simulink model "BlsmControl_color"  (R2014a)
settings: Solver=FixedStepDiscrete  SolverMode=SingleTasking  StartTime=0.0  StopTime=6  FixedStep=1e-4  MinStep=1e-7  RelTol=1e-4  AbsTol=1e-4
PostLoadFcn:
  | parameter
InitFcn:
  | parameter
undefined symbols (not defined in the file): PI, rpm_ast
libraries: simulink x1
settings Model: CovSFcnEnable=on  ExtModeTrigDuration=100  BufferReuse=off  Creator=matsumoto  LastModifiedBy=ts1413
settings DataIOCC: SaveFinalState=on  SignalLoggingSaveFormat=ModelDataLogs  SaveOutput=off  SaveState=on  StateSaveName=tmp_raccel_xout  SignalLoggingName=tmp_raccel_logsout
settings OptimizationCC: BlockReduction=off  OptimizeBlockIOStorage=off  BufferReuse=off  GlobalBufferReuse=off  ExpressionFolding=off  ExpressionDepthLimit=2147483647  LocalBlockOutputs=off  EfficientMapNaN2IntZero=off  OptimizeModelRefInitCode=on  LifeSpan=1
settings DebuggingCC: ConsistencyChecking=warning  UnderspecifiedInitializationDetection=Classic  TimeAdjustmentMsg=warning  FcnCallInpInsideContextMsg=UseLocalSettings  FrameProcessingCompatibilityMsg=error  StateNameClashWarn=warning
settings HardwareCC: TargetBitPerLong=64  TargetBitPerPointer=64  TargetLongLongMode=on  TargetIntDivRoundTo=Zero  TargetEndianess=LittleEndian  TargetWordSize=64  TargetHWDeviceType=MATLAB Host  ProdEqTarget=off
settings RTWCC: SystemTargetFile=ert.tlc  GenCodeOnly=on  TemplateMakefile=ert_default_tmf  Description=Embedded Coder  ProcessScript=ert_make_rtw_hook
settings CodeAppCC: IgnoreCustomStorageClasses=off  MaxIdLength=128
settings ERTTargetCC: ParMdlRefBuildCompliant=on  CompOptLevelCompliant=on  ConcurrentExecutionCompliant=on  ERTFirstTimeCompliant=on  ModelStepFunctionPrototypeControlCompliant=on  CPPClassGenCompliant=on  InlinedParameterPlacement=Hierarchical  ERTCustomFileTemplate=example_file_process.tlc
settings ConfigComp: CovMetricSettings=dw  CovHtmlReporting=on  CovSaveCumulativeToWorkspaceVar=on  CovSaveSingleToWorkspaceVar=on  CovModelRefEnable=Off  CovExternalEMLEnable=off

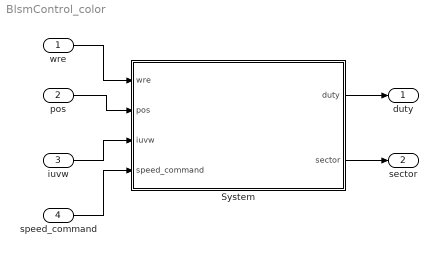
== system BlsmControl_color ==
  wre : Inport
  pos : Inport  Port=2
  iuvw : Inport  Port=3
  speed_command : Inport  Port=4
  System : Subsystem
  duty : Outport
  sector : Outport  Port=2
  wires:
  wre/1 -> System/1(wre)
  pos/1 -> System/2(pos)
  iuvw/1 -> System/3(iuvw)
  speed_command/1 -> System/4(speed_command)
  System/1(duty) -> duty/1
  System/2(sector) -> sector/1

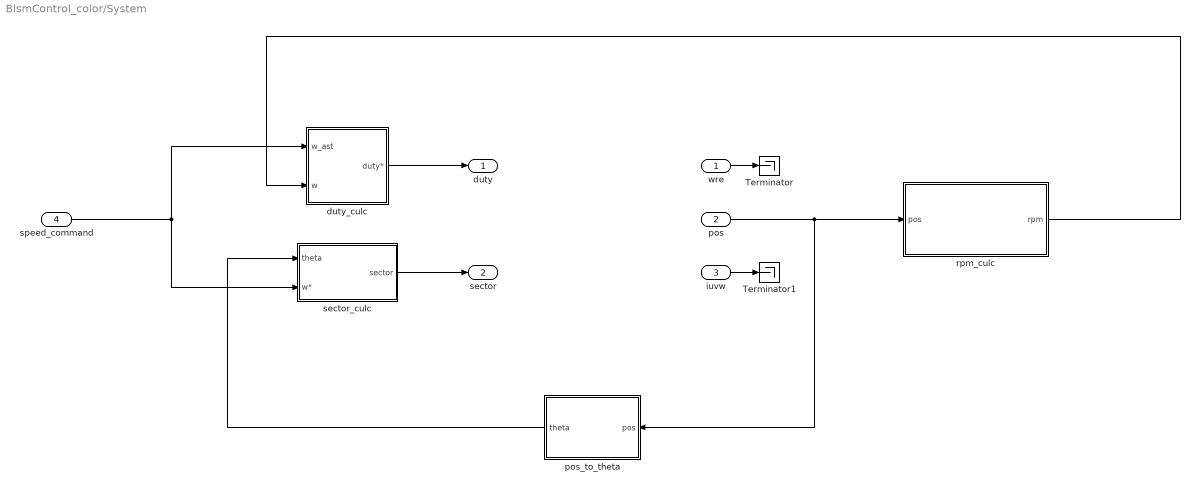
== system BlsmControl_color/System ==
  wre : Inport
  pos : Inport  Port=2
  iuvw : Inport  Port=3
  speed_command : Inport  Port=4
  Terminator : Terminator
  Terminator1 : Terminator
  duty_culc : Subsystem
  pos_to_theta : Subsystem
  rpm_culc : Subsystem
  sector_culc : Subsystem
  duty : Outport
  sector : Outport  Port=2
  wires:
  sector_culc/1(sector) -> sector/1
  pos/1 -> rpm_culc/1(pos), pos_to_theta/1(pos)
  duty_culc/1(duty*) -> duty/1
  speed_command/1 -> duty_culc/1(w_ast), sector_culc/2(w*)
  rpm_culc/1(rpm) -> duty_culc/2(w)
  wre/1 -> Terminator/1
  iuvw/1 -> Terminator1/1
  pos_to_theta/1("theta ") -> sector_culc/1(theta)

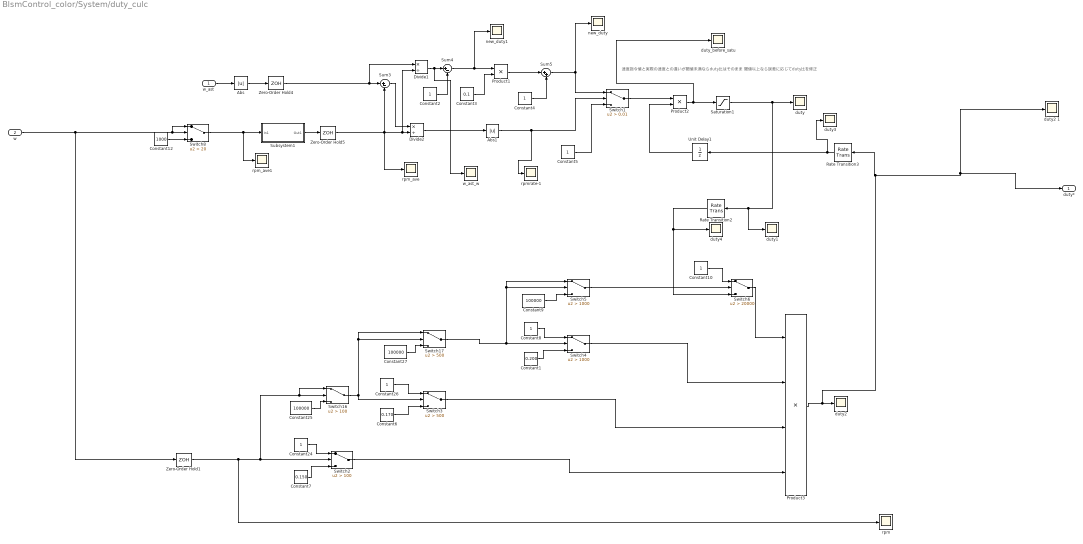
== system BlsmControl_color/System/duty_culc ==
  note: 速度指令値と実際の速度との違いが閾値未満ならduty比はそのまま
      | 閾値以上なら誤差に応じてduty比を修正
  w_ast : Inport
  w : Inport  Port=2
  Abs : Abs
  Abs1 : Abs
  Constant1 : Constant  Value=0.200
  Constant{2,4..5,8,10,24,26} (7 alike) : Constant
  Constant12 : Constant  Value=1000
  Constant25 : Constant  Value=100000
  Constant27 : Constant  Value=100000
  Constant3 : Constant  Value=0.1
  Constant6 : Constant  Value=0.170
  Constant7 : Constant  Value=0.150
  Constant9 : Constant  Value=100000
  Divide1 : Product  Inputs=*/
  Divide2 : Product  Inputs=*/
  Product1 : Product
  Product2 : Product
  Product3 : Product  Inputs=4
  Rate Transition2 : RateTransition  Integrity=off  OutPortSampleTime=1e-4
  Rate Transition3 : RateTransition  OutPortSampleTime=1e-2
  Saturation1 : Saturate  UpperLimit=1  LowerLimit=0
  Subsystem1 : Subsystem
  Sum3 : Sum  Inputs=|+-
  Sum4 : Sum  Inputs=|+-
  Sum5 : Sum  Inputs=|++
  Switch1 : Switch  Criteria=u2 > Threshold  Threshold=0.01
  Switch16 : Switch  Criteria=u2 > Threshold  Threshold=100
  Switch17 : Switch  Criteria=u2 > Threshold  Threshold=500
  Switch2 : Switch  Criteria=u2 > Threshold  Threshold=100
  Switch3 : Switch  Criteria=u2 > Threshold  Threshold=500
  Switch4 : Switch  Criteria=u2 > Threshold  Threshold=1000
  Switch5 : Switch  Criteria=u2 > Threshold  Threshold=1000
  Switch6 : Switch  Criteria=u2 > Threshold  Threshold=20000
  Switch8 : Switch  Criteria=u2 > Threshold  Threshold=20
  Unit Delay1 : UnitDelay  SampleTime=1e-2
  Zero-Order Hold1 : ZeroOrderHold  SampleTime=1e-4
  Zero-Order Hold4 : ZeroOrderHold  SampleTime=1e-2
  Zero-Order Hold5 : ZeroOrderHold  SampleTime=1e-2
  duty{,1,3..4} (4 alike) : Scope
      duty settings: YMin=-0.05428  YMax=0.48851  SaveName=ScopeData2
      duty1 settings: YMin=-0.125  YMax=1.125
      duty3 settings: YMin=0.1347  YMax=0.17568
      duty4 settings: YMin=-0.125  YMax=1.125  SaveName=ScopeData2
  "duty2 " : Scope
      settings: YMin=-0.05313  YMax=0.47817
  duty2 1 : Scope
      settings: YMin=-0.125  YMax=1.125  SaveName=ScopeData3
  duty_before_satu : Scope
      settings: YMin=-15.2255  YMax=43.91394  SaveName=ScopeData3
  new_duty : Scope
      settings: YMin=-1.50812  YMax=1.82498  SaveName=ScopeData7
  new_duty1 : Scope
      settings: YMin=-376.00000  YMax=3374.00000  SaveName=ScopeData3
  "rpm " : Scope
      settings: YMin=-355.87867  YMax=3202.908
  rpm_ave : Scope
      settings: YMin=-1366.39339  YMax=12497.5005  SaveName=ScopeData3
  rpm_ave1 : Scope
      settings: YMin=-5.29357  YMax=8.40286  SaveName=ScopeData5
  rpmrate-1 : Scope
      settings: YMin=-0.28  YMax=2.92  SaveName=ScopeData3
  w_ast_w : Scope
      settings: YMin=-375.00000  YMax=3375.00000  SaveName=ScopeData4
  duty* : Outport
  wires:
  Constant2/1 -> Sum4/2
  Sum4/1 -> new_duty1/1, Product1/1
  Constant3/1 -> Product1/2
  Product1/1 -> Sum5/1
  Constant4/1 -> Sum5/2
  Sum3/1 -> Divide2/1
  Divide1/1 -> w_ast_w/1, Sum4/1
  Divide2/1 -> Abs1/1
  Constant5/1 -> Switch1/3
  Abs1/1 -> rpmrate-1/1, Switch1/2
  Unit Delay1/1 -> Product2/2
  w_ast/1 -> Abs/1
  Sum5/1 -> new_duty/1, Switch1/1
  Constant1/1 -> Switch4/3
  Constant6/1 -> Switch3/3
  Constant7/1 -> Switch2/3
  Constant24/1 -> Switch2/1
  Constant25/1 -> Switch16/3
  Constant26/1 -> Switch3/1
  Constant27/1 -> Switch17/3
  Switch16/1 -> Switch3/2, Switch17/1, Switch17/2
  Switch17/1 -> Switch5/1, Switch5/2, Switch4/2
  Constant8/1 -> Switch4/1
  Constant9/1 -> Switch5/3
  Constant10/1 -> Switch6/1
  Switch6/1 -> Product3/1
  Product2/1 -> Saturation1/1, duty_before_satu/1
  Saturation1/1 -> Rate Transition2/1, duty1/1, duty/1
  Switch4/1 -> Product3/2
  Switch3/1 -> Product3/3
  Switch2/1 -> Product3/4
  Switch5/1 -> Switch6/2
  Subsystem1/1(Out1) -> Zero-Order Hold5/1
  Zero-Order Hold4/1 -> Divide1/1, Sum3/1
  Zero-Order Hold1/1 -> "rpm "/1, Switch16/1, Switch16/2, Switch2/2
  Zero-Order Hold5/1 -> rpm_ave/1, Sum3/2, Divide1/2, Divide2/2
  Switch1/1 -> Product2/1
  Rate Transition2/1 -> duty4/1, Switch6/3
  Rate Transition3/1 -> Unit Delay1/1, duty3/1
  Switch8/1 -> rpm_ave1/1, Subsystem1/1(In1)
  Constant12/1 -> Switch8/3
  Product3/1 -> duty*/1, duty2 1/1, Rate Transition3/1, "duty2 "/1
  w/1 -> Switch8/2, Switch8/1, Zero-Order Hold1/1
  Abs/1 -> Zero-Order Hold4/1

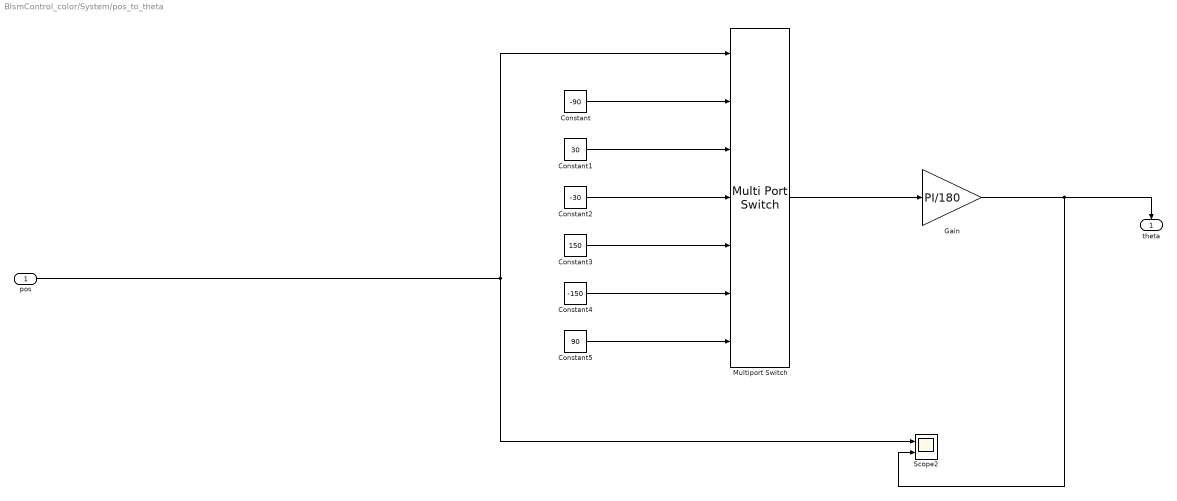
== system BlsmControl_color/System/pos_to_theta ==
  pos : Inport
  Constant : Constant  Value=-90
  Constant1 : Constant  Value=30
  Constant2 : Constant  Value=-30
  Constant3 : Constant  Value=150
  Constant4 : Constant  Value=-150
  Constant5 : Constant  Value=90
  Gain : Gain  Gain=PI/180
  Multiport Switch : MultiPortSwitch  DataPortOrder=Specify indices  Inputs=6  DataPortIndices={1,2,3,4,5,6}
  Scope2 : Scope  NumInputPorts=2
      settings: YMin=-224.98722~-0.625  YMax=224.98648~5.625  SaveName=ScopeData4
  "theta " : Outport
  wires:
  pos/1 -> Multiport Switch/1, Scope2/1
  Constant/1 -> Multiport Switch/2
  Constant1/1 -> Multiport Switch/3
  Constant2/1 -> Multiport Switch/4
  Constant5/1 -> Multiport Switch/7
  Constant4/1 -> Multiport Switch/6
  Constant3/1 -> Multiport Switch/5
  Multiport Switch/1 -> Gain/1
  Gain/1 -> Scope2/2, "theta "/1

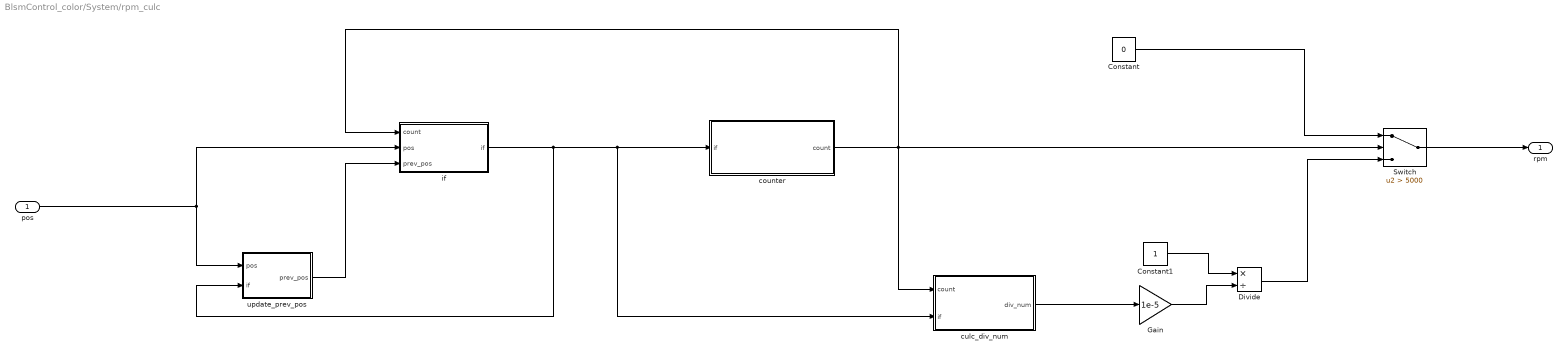
== system BlsmControl_color/System/rpm_culc ==
  pos : Inport
  Constant : Constant  Value=0
  Constant1 : Constant
  Divide : Product  Inputs=*/
  Gain : Gain  Gain=1e-5
  Switch : Switch  Criteria=u2 > Threshold  Threshold=5000
  counter : Subsystem
  culc_div_num : Subsystem
  if : Subsystem
  update_prev_pos : Subsystem
  rpm : Outport
  wires:
  pos/1 -> if/2(pos), update_prev_pos/1(pos)
  culc_div_num/1(div_num) -> Gain/1
  Gain/1 -> Divide/2
  Constant1/1 -> Divide/1
  Divide/1 -> Switch/3
  Constant/1 -> Switch/1
  Switch/1 -> rpm/1
  counter/1(count) -> culc_div_num/1(count), if/1(count), Switch/2
  if/1(if) -> counter/1(if), culc_div_num/2(if), update_prev_pos/2(if)
  update_prev_pos/1(prev_pos) -> if/3(prev_pos)

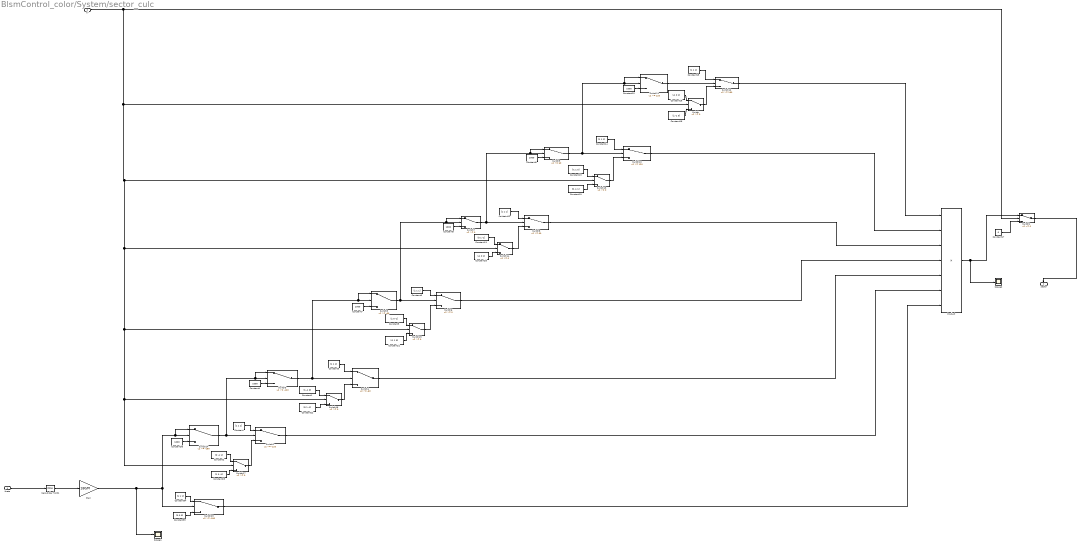
== system BlsmControl_color/System/sector_culc ==
  theta : Inport
  w* : Inport  Port=2
  Constant{,3,6,12,14..15,34} (7 alike) : Constant  Value=[1 1 1]
  Constant1 : Constant  Value=[1 -1 0]
  Constant{4,7..10,36} (6 alike) : Constant  Value=1000
  Constant11 : Constant  Value=[0 1 -1]
  Constant13 : Constant  Value=[-1 1 0]
  Constant16 : Constant  Value=[-1 0 1]
  Constant17 : Constant  Value=0
  Constant18 : Constant  Value=[1 -1 0]
  Constant19 : Constant  Value=[0 -1 1]
  Constant2 : Constant  Value=[0 -1 1]
  Constant20 : Constant  Value=[-1 0 1]
  Constant21 : Constant  Value=[-1 1 0]
  Constant22 : Constant  Value=[0 1 -1]
  Constant23 : Constant  Value=[1 0 -1]
  Constant35 : Constant  Value=[0 0 0]
  Constant5 : Constant  Value=[1 0 -1]
  Gain : Gain  Gain=180/PI
  Product : Product  Inputs=7
  Scope1 : Scope
      settings: YMin=-224.986  YMax=224.99544
  Scope2 : Scope
      settings: YMin=-1  YMax=1  SaveName=ScopeData4
  Switch{,6..7,13..17} (8 alike) : Switch
  Switch1 : Switch  Criteria=u2 ~= 0
  Switch10 : Switch  Threshold=120
  Switch11 : Switch  Threshold=120
  Switch12 : Switch  Threshold=180
  Switch2 : Switch  Threshold=-120
  Switch23 : Switch  Threshold=-180
  Switch24 : Switch  Threshold=-180
  Switch3 : Switch  Threshold=-120
  Switch4 : Switch  Threshold=-60
  Switch5 : Switch  Threshold=-60
  Switch8 : Switch  Threshold=60
  Switch9 : Switch  Threshold=60
  Zero-Order Hold1 : ZeroOrderHold  SampleTime=1e-4
  sector : Outport
  wires:
  Constant/1 -> Switch2/1
  Constant12/1 -> Switch8/1
  Switch10/1 -> Product/2
  Switch2/1 -> Product/6
  Switch/1 -> Switch12/3
  Switch7/1 -> Switch9/2, Switch9/1, Switch8/2
  Switch8/1 -> Product/3
  Constant7/1 -> Switch5/3
  Constant4/1 -> Switch3/3
  Constant10/1 -> Switch11/3
  Switch6/1 -> Product/4
  Constant11/1 -> Switch14/1
  Constant6/1 -> Switch6/1
  Constant8/1 -> Switch7/3
  Constant9/1 -> Switch9/3
  Constant13/1 -> Switch13/1
  Constant14/1 -> Switch10/1
  Constant15/1 -> Switch12/1
  Constant2/1 -> Switch17/1
  Constant3/1 -> Switch4/1
  Switch3/1 -> Switch5/1, Switch5/2, Switch4/2
  Switch11/1 -> Switch12/2
  Switch12/1 -> Product/1
  Switch4/1 -> Product/5
  Switch5/1 -> Switch6/2, Switch7/2, Switch7/1
  Constant1/1 -> Switch16/1
  Switch9/1 -> Switch11/1, Switch11/2, Switch10/2
  theta/1 -> Zero-Order Hold1/1
  Switch24/1 -> Switch3/1, Switch3/2, Switch2/2
  Zero-Order Hold1/1 -> Gain/1
  Constant34/1 -> Switch23/1
  Constant36/1 -> Switch24/3
  Constant35/1 -> Switch23/3
  Switch23/1 -> Product/7
  Gain/1 -> Switch24/1, Switch24/2, Switch23/2, Scope1/1
  Product/1 -> Scope2/1, Switch1/1
  w*/1 -> Switch1/2, Switch/2, Switch13/2, Switch14/2, Switch15/2, Switch17/2, Switch16/2
  Constant17/1 -> Switch1/3
  Switch1/1 -> sector/1
  Constant16/1 -> Switch/1
  Switch13/1 -> Switch10/3
  Constant18/1 -> Switch/3
  Constant19/1 -> Switch13/3
  Switch14/1 -> Switch8/3
  Constant20/1 -> Switch14/3
  Switch15/1 -> Switch6/3
  Constant5/1 -> Switch15/1
  Constant21/1 -> Switch15/3
  Switch16/1 -> Switch4/3
  Constant22/1 -> Switch16/3
  Switch17/1 -> Switch2/3
  Constant23/1 -> Switch17/3

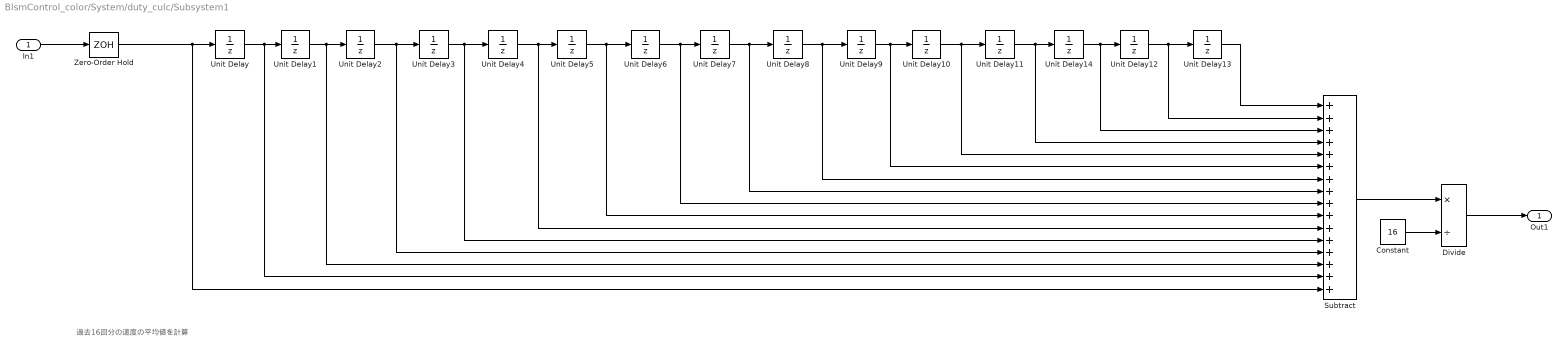
== system BlsmControl_color/System/duty_culc/Subsystem1 ==
  note: 過去16回分の速度の平均値を計算
  In1 : Inport
  Constant : Constant  Value=16
  Divide : Product  Inputs=*/
  Subtract : Sum  Inputs=++++++++++++++++
  Unit Delay{,1..14} (15 alike) : UnitDelay  InitialCondition=rpm_ast  SampleTime=-1
  Zero-Order Hold : ZeroOrderHold  SampleTime=1e-4
  Out1 : Outport
  wires:
  Divide/1 -> Out1/1
  Constant/1 -> Divide/2
  Subtract/1 -> Divide/1
  In1/1 -> Zero-Order Hold/1
  Unit Delay5/1 -> Unit Delay6/1, Subtract/10
  Unit Delay8/1 -> Unit Delay9/1, Subtract/7
  Unit Delay10/1 -> Unit Delay11/1, Subtract/5
  Unit Delay9/1 -> Unit Delay10/1, Subtract/6
  Unit Delay7/1 -> Unit Delay8/1, Subtract/8
  Unit Delay6/1 -> Subtract/9, Unit Delay7/1
  Unit Delay4/1 -> Unit Delay5/1, Subtract/11
  Unit Delay2/1 -> Unit Delay3/1, Subtract/13
  Unit Delay3/1 -> Unit Delay4/1, Subtract/12
  Unit Delay11/1 -> Unit Delay14/1, Subtract/4
  Unit Delay12/1 -> Unit Delay13/1, Subtract/2
  Unit Delay14/1 -> Unit Delay12/1, Subtract/3
  Unit Delay13/1 -> Subtract/1
  Unit Delay/1 -> Unit Delay1/1, Subtract/15
  Unit Delay1/1 -> Unit Delay2/1, Subtract/14
  Zero-Order Hold/1 -> Unit Delay/1, Subtract/16

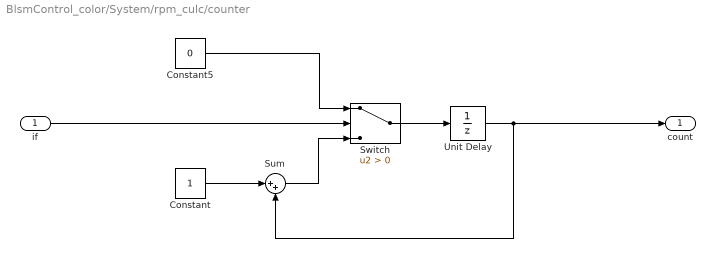
== system BlsmControl_color/System/rpm_culc/counter ==
  if : Inport
  Constant : Constant
  Constant5 : Constant  Value=0
  Sum : Sum  Inputs=|++
  Switch : Switch  Criteria=u2 > Threshold
  Unit Delay : UnitDelay  InitialCondition=5001  SampleTime=-1
  count : Outport
  wires:
  if/1 -> Switch/2
  Switch/1 -> Unit Delay/1
  Unit Delay/1 -> Sum/2, count/1
  Constant/1 -> Sum/1
  Constant5/1 -> Switch/1
  Sum/1 -> Switch/3

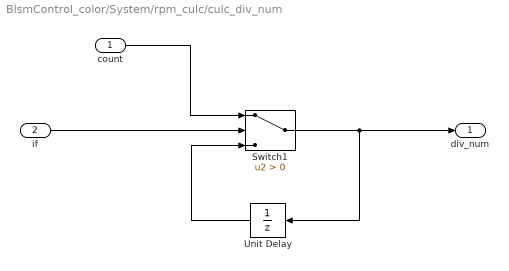
== system BlsmControl_color/System/rpm_culc/culc_div_num ==
  count : Inport
  if : Inport  Port=2
  Switch1 : Switch  Criteria=u2 > Threshold
  Unit Delay : UnitDelay  InitialCondition=5001  SampleTime=-1
  div_num : Outport
  wires:
  Unit Delay/1 -> Switch1/3
  Switch1/1 -> div_num/1, Unit Delay/1
  if/1 -> Switch1/2
  count/1 -> Switch1/1

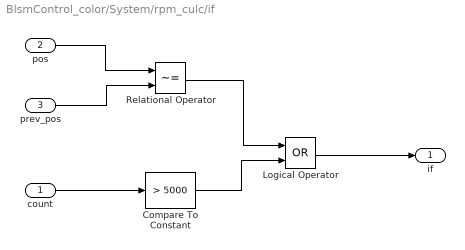
== system BlsmControl_color/System/rpm_culc/if ==
  count : Inport
  pos : Inport  Port=2
  prev_pos : Inport  Port=3
  Compare To Constant : simulink/Logic and Bit Operations/Compare To Constant  relop=>  const=5000  OutDataTypeStr=boolean
  Logical Operator : Logic  Operator=OR  AllPortsSameDT=off  OutDataTypeStr=boolean
  Relational Operator : RelationalOperator  Operator=~=  OutDataTypeStr=boolean
  if : Outport
  wires:
  pos/1 -> Relational Operator/1
  count/1 -> Compare To Constant/1
  Relational Operator/1 -> Logical Operator/1
  Compare To Constant/1 -> Logical Operator/2
  prev_pos/1 -> Relational Operator/2
  Logical Operator/1 -> if/1

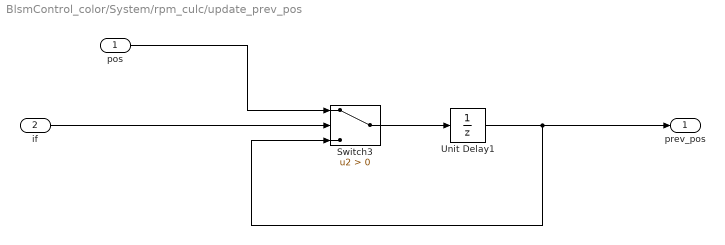
== system BlsmControl_color/System/rpm_culc/update_prev_pos ==
  pos : Inport
  if : Inport  Port=2
  Switch3 : Switch  Criteria=u2 > Threshold
  Unit Delay1 : UnitDelay  InitialCondition=5001  SampleTime=-1
  prev_pos : Outport
  wires:
  if/1 -> Switch3/2
  Unit Delay1/1 -> Switch3/3, prev_pos/1
  pos/1 -> Switch3/1
  Switch3/1 -> Unit Delay1/1
